simulink model "chap11_6sim"  (R2023b)
settings: Solver=ode45  StartTime=0.0  StopTime=10  RelTol=1e-3
values from neighbouring files (symbols this model uses):
  b = 1    [chap11_4int.m]    (also in chap11_6int.m = 0.5)
  f1 = b + kd * kv    (= 12.5)    [chap11_6int.m]
  f2 = J    (= 2)    [chap11_6int.m]
  J = 1.0    (= 1)    [chap11_1plant.m]    (also in chap11_4int.m = 2; chap11_6int.m = 2)
  kd = 6    [chap11_4int.m]    (also in chap11_6int.m)
  kp = 15    [chap11_6int.m]
  kv = 2    [chap11_4int.m]    (also in chap11_6int.m)
settings Model: Creator=CorgiQvm  LastModifiedBy=CorgiQvm
settings DataIOCC: SaveFormat=Array  ReturnWorkspaceOutputs=off
settings ModelReferenceCC: PropagateSignalLabelsOutOfModel=off

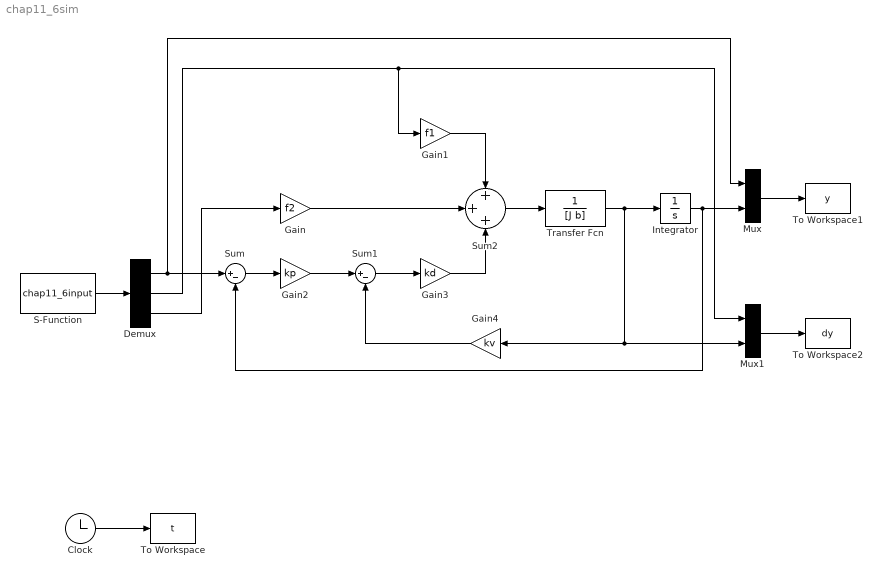
== system chap11_6sim ==
  Clock : Clock
  Demux : Demux  Outputs=3
      settings: DisplayOption=none
  Gain : Gain  Gain=f2  OutDataTypeStr=Inherit: Same as input
  Gain1 : Gain  Gain=f1  OutDataTypeStr=Inherit: Same as input
  Gain2 : Gain  Gain=kp  OutDataTypeStr=Inherit: Same as input
  Gain3 : Gain  Gain=kd  OutDataTypeStr=Inherit: Same as input
  Gain4 : Gain  Gain=kv  OutDataTypeStr=Inherit: Same as input
  Integrator : Integrator
  Mux : Mux  Inputs=2
  Mux1 : Mux  Inputs=2
  S-Function : S-Function  FunctionName=chap11_6input  SFunctionDeploymentMode=off  EnableBusSupport=off
  Sum : Sum  Inputs=|+-  InputSameDT=on  SaturateOnIntegerOverflow=on  OutDataTypeStr=Inherit: Same as first input
  Sum1 : Sum  Inputs=|+-  InputSameDT=on  SaturateOnIntegerOverflow=on  OutDataTypeStr=Inherit: Same as first input
  Sum2 : Sum  Inputs=+++  InputSameDT=on  SaturateOnIntegerOverflow=on  OutDataTypeStr=Inherit: Same as first input
  To Workspace : ToWorkspace  VariableName=t  SampleTime=-1
  To Workspace1 : ToWorkspace  VariableName=y  SampleTime=-1
  To Workspace2 : ToWorkspace  VariableName=dy  SampleTime=-1
  Transfer Fcn : TransferFcn  Denominator=[J b]
  wires:
  Clock/1 -> To Workspace/1
  S-Function/1 -> Demux/1
  Demux/1 -> Mux/1, Sum/1
  Sum/1 -> Gain2/1
  Gain2/1 -> Sum1/1
  Sum1/1 -> Gain3/1
  Gain3/1 -> Sum2/3
  Sum2/1 -> Transfer Fcn/1
  Transfer Fcn/1 -> Mux1/2, Gain4/1, Integrator/1
  Integrator/1 -> Sum/2, Mux/2
  Mux/1 -> To Workspace1/1
  Gain4/1 -> Sum1/2
  Mux1/1 -> To Workspace2/1
  Demux/2 -> Gain1/1, Mux1/1
  Gain1/1 -> Sum2/1
  Gain/1 -> Sum2/2
  Demux/3 -> Gain/1
